simulink model "fft32kpt_ssr16_fixed"  (R2024b)
settings: Solver=VariableStepAuto  StartTime=0.0  StopTime=sample_period*N*5  RelTol=1e-3
PreLoadFcn:
  | clk_freq = 570e6; % PL clock frequency
  | sample_period = 1/(570e6*16); % 570Msps*16parallel paths
  | N=32768; % fft point size
  | binw=(1/sample_period) / 2*N; % bin width
  | 
  | bin_freq = 2*pi*11*binw+pi*binw; % sin, cos freq centering per channel
  | 
  | % for transpose block
  | DATA_WIDTH=16;
  | SSR=16;
  | M=16;
  | N1=N/M;
  | MEM_STYLE=4; % MEM OPTIONS: 4 - ULTRA, 0 - AUTO, 1 - BRAM, 5 - MIXED
InitFcn:
  | clk_freq = 570e6; % PL clock frequency
  | sample_period = 1/(570e6*16); % 570Msps*16parallel paths
  | N=32768; % fft point size
  | binw=(1/sample_period) / 2*N; % bin width
  | 
  | bin_freq = 2*pi*11*binw+pi*binw; % sin, cos freq centering per channel
  | 
  | % for transpose block
  | DATA_WIDTH=16;
  | SSR=16;
  | M=16;
  | N1=N/M;
  | MEM_STYLE=4; % MEM OPTIONS: 4 - ULTRA, 0 - AUTO, 1 - BRAM, 5 - MIXED
undefined symbols (not defined in the file or in its folder): None, S, vsva2197, xcvc1902
libraries: aieBasic x47, hdlBasic x39, aieUtilities x16, aieDSP x16, hdlUtilities x16, matrix_library x16, hdlSSR x13, simulink x1, dspxfrm3 x1, vmcUtilities x1
(part 1 of 3)
settings Model: Creator=mmi  LastModifiedBy=robg
settings DebuggingCC: UnconnectedInputMsg=warning  UnconnectedOutputMsg=warning  UnconnectedLineMsg=warning
settings HardwareCC: ProdBitPerPointer=32  ProdBitPerSizeT=32  ProdBitPerPtrDiffT=32  ProdLargestAtomicFloat=None  ProdIntDivRoundTo=Undefined  ProdEndianess=Unspecified  ProdWordSize=32  ProdHWDeviceType=ASIC/FPGA->ASIC/FPGA  TargetBitPerLong=64  TargetBitPerPointer=64  TargetBitPerSizeT=64  TargetBitPerPtrDiffT=64  TargetLongLongMode=on  TargetIntDivRoundTo=Zero  TargetEndianess=LittleEndian  TargetWordSize=64  TargetHWDeviceType=Custom Processor->MATLAB Host Computer  ProdEqTarget=off
settings ModelReferenceCC: EnableRefExpFcnMdlSchedulingChecks=on
settings RTWCC: GPUComputeCapability=3.5  DLArmComputeVersion=19.05
settings ConfigComp: CovBoundaryAbsTol=1.0e-5

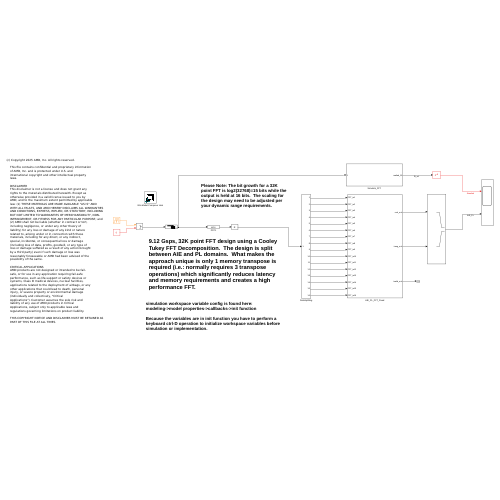
[thumbnail: Simulink's stored preview of the top-level diagram]
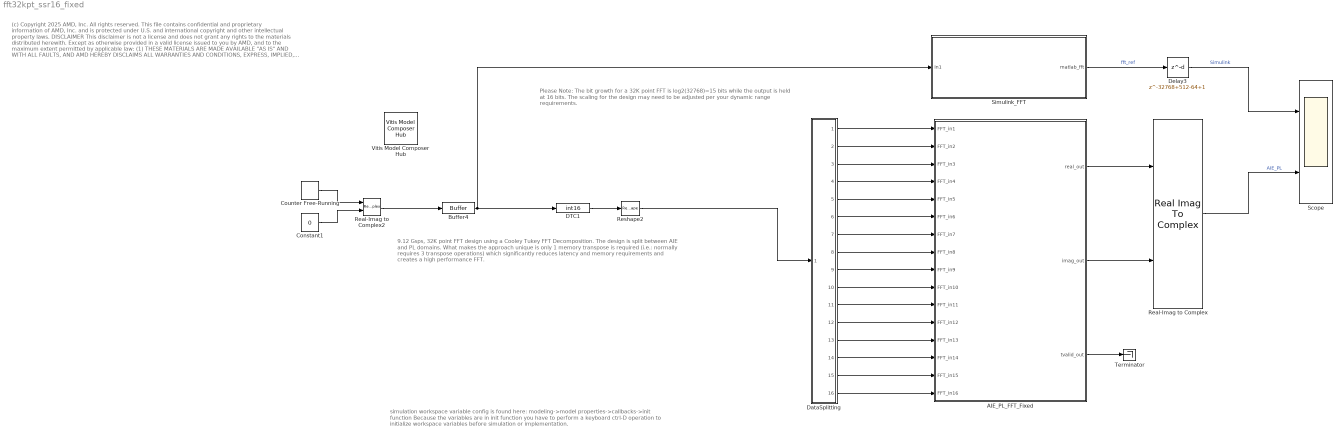
== system fft32kpt_ssr16_fixed ==
  note: simulation workspace variable config is found here:
      | modeling->model properties->callbacks->init function
      |
      | Because the variables are in init function you have to perform a keyboard ctrl-D operation to initialize workspace variables before simulation or implementation.
  note: 9.12 Gsps, 32K point FFT design using a Cooley Tukey FFT Decomposition. The design is split between AIE and PL domains. What makes the approach unique is only 1 memory transpose is required (i.e.: normally requires 3 transpose operations) which significantly reduces latency and memory requirements and creates a high performance FFT.
  note: Please Note: The bit growth for a 32K point FFT is log2(32768)=15 bits while the output is held at 16 bits. The scaling for the design may need to be adjusted per your dynamic range requirements.
  note: (c) Copyright 2025 AMD, Inc. All rights reserved.
      |
      | This file contains confidential and proprietary information
      | of AMD, Inc. and is protected under U.S. and
      | international copyright and other intellectual property
      | laws.
      |
      | DISCLAIMER
      | This disclaimer is not a license and does not grant any
      | rights to the materials distributed herewith. Except as
      | otherwise provided in a valid license issued to you by
      | AMD, and to the maximum extent permitted by applicable
      | law: (1) THESE MATERIALS ARE MADE AVAILABLE "AS IS" AND
      | WITH ALL FAULTS, AND AMD HEREBY DISCLAIMS ALL WARRANTIES
      | AND CONDITIONS, EXPRESS, IMPLIED, OR STATUTORY, INCLUDING
      | BUT NOT LIMITED TO WARRANTIES OF MERCHANTABILITY, NON-
      | INFRINGEMENT, OR FITNESS FOR ANY PARTICULAR PURPOSE; and
      | (2) AMD shall not be liable (whether in contract or tort,
      | including negligence, or under any other theory of
      | liability) for any loss or damage of any kind or nature
      | related to, arising under or in connection with these
      | materials, including for any direct, or any indirect,
      | special, incidental, or consequential loss or damage
      | (including loss of data, profits, goodwill, or any type of
      | loss or damage suffered as a result of any action brought
      | by a third party) even if such damage or loss was
      | reasonably foreseeable or AMD had been advised of the
      | possibility of the same.
      |
      | CRITICAL APPLICATIONS
      | AMD products are not designed or intended to be fail-
      | safe, or for use in any application requiring fail-safe
      | performance, such as life-support or safety devices or
      | systems, Class III medical devices, nuclear facilities,
      | applications related to the deployment of airbags, or any
      | other applications that could lead to death, personal
      | injury, or severe property or environmental damage
      | (individually and collectively, "Critical
      | Applications"). Customer assumes the sole risk and
      | liability of any use of AMD products in Critical
      | Applications, subject only to applicable laws and
      | regulations governing limitations on product liability.
      |
      | THIS COPYRIGHT NOTICE AND DISCLAIMER MUST BE RETAINED AS
      | PART OF THIS FILE AT ALL TIMES.
  AIE_PL_FFT_Fixed : Subsystem
  Buffer4 : Buffer  N=N  OutputFrames=off
  Constant1 : Constant  Value=0  OutDataTypeStr=Inherit: Inherit via back propagation  SampleTime=sample_period
  Counter Free-Running : simulink/Sources/Counter Free-Running  NumBits=log2(1024)  tsamp=sample_period
  DTC1 : DataTypeConversion  OutDataTypeStr=int16  SaturateOnIntegerOverflow=off  RndMeth=Floor
  DataSplitting : Subsystem
  Delay3 : Delay  DelayLength=32768+512-64+1
  Real-Imag to Complex : RealImagToComplex
  Real-Imag to Complex2 : RealImagToComplex
  Reshape2 : Reshape  OutputDimensionality=Customize  OutputDimensions=[16,N/16]
  Scope : Scope  NumInputPorts=2
  Simulink_FFT : Subsystem
  Terminator : Terminator
  Vitis Model Composer Hub : vmcUtilities/Vitis Model Composer Hub  Tag=genX  CodeGeneration=off  SubsystemName=AIE_2kFFT_cplxRot  BlockHierPath=fft32kpt_ssr16_fixed/AIE_PL_FFT_Fixed/AIE_2kFFT_cplxRot  CompilationType=VitisCompilation  SubsystemType=AIENode  ExportTypeV2=GenXO  StartColumn=1  NumberOfColumns=1  TargetDirectory=./code_FFT  exportDesign=off  analyzeDesign=on  validateDesignOnHw=off  ExportType=Vitis Subsystem  IpVendor=xilinx.com  IpLibrary=hls  IpVersion=1.0  IpHWLanguage=Verilog  AieCompilerOptions={}  AieSimulatorOptions={}  CreateTestbench=on  TestbenchStackSize=10  RunRtlSim=off  RunCSim=off  RunAieSim=on  AieSimTimeout=50000  RunAieSimProfiling=off  LaunchVitisAnalyzer=off  PlotOutput=off  RunX86Sim=off  X86SimTimeout=10  GenHwImage=off  GenLibadfXo=off  GenHwValidationCode=off  PlatformType=Specify Platform  Platform=/proj/xbuilds/SWIP/2024.2_1113_1001/installs/lin64/Vitis/2024.2/base_platforms/xilinx_vck190_base_202420_1/xilinx_vck190_base_202420_1.xpfm  HwSystemType=Baremetal  HwValidationTarget=hw  ProjDevice=Versal VCK190 Evaluation Platform (xcvc1902-vsva2197-2MP-e-S)  ProjDevicePart=xcvc1902-vsva2197-2MP-e-S  AIEType=AIE  SamplePeriod=-1  ClockFrequency=200  DataPathParallelism=1  xilinxfamily=versalaicore  part=xcvc1902  speed=-2MP-e-S  package=vsva2197  directory=./netlist_pl/ip/HDL_16ptFFT_tranpose/src  testbench=off  incr_netlist=off  synthesis_tool=Vivado  clock_wrapper=Clock Enables  dbl_ovrd=According to Block Masks  dcm_input_clock_period=10  sysclk_period=1e9/clk_freq  simulink_period=1/clk_freq  eval_field=0  IPInfoJsonString="{\"DUTSubsystemName\":\"AIE_2kFFT_cplxRot\",\"AIESubsystem\":{\"SubsystemName\":\"AIE_2kFFT_cplxRot\",\"TargetDirectory\":\"./code_FFT\",\"AIEArrayConfig\":\"Use entire AIE array\",\"StartColumn\":\"0\",\"NumberOfColumns\":\"1\"},\"SubsystemTag\":\"AIENode\"}"  LogFileName=/group/xcoswmktg2/robg/git/vmc_examples/github/Examples/AIENGINE_plus_PL/AIE_HDL/VersalFFT/code_FFT/model_composer.log  NThreads=4  IPConfigFile=/tmp/vmctmp-16428498816969006604/fft32kpt_ssr16_fixed_ipconfig.json
  wires:
  Buffer4/1 -> Simulink_FFT/1(In1), DTC1/1
  Constant1/1 -> Real-Imag to Complex2/2
  Counter Free-Running/1 -> Real-Imag to Complex2/1
  Real-Imag to Complex2/1 -> Buffer4/1
  DTC1/1 -> Reshape2/1
  Simulink_FFT/1(matlab_fft) -> Delay3/1  "fft_ref"
  Delay3/1 -> Scope/1  "Simulink"
  Reshape2/1 -> DataSplitting/1(In1)
  DataSplitting/1(Out1) -> AIE_PL_FFT_Fixed/1(FFT_in1)
  DataSplitting/2(Out2) -> AIE_PL_FFT_Fixed/2(FFT_in2)
  DataSplitting/3(Out3) -> AIE_PL_FFT_Fixed/3(FFT_in3)
  DataSplitting/4(Out4) -> AIE_PL_FFT_Fixed/4(FFT_in4)
  DataSplitting/5(Out5) -> AIE_PL_FFT_Fixed/5(FFT_in5)
  DataSplitting/6(Out6) -> AIE_PL_FFT_Fixed/6(FFT_in6)
  DataSplitting/7(Out7) -> AIE_PL_FFT_Fixed/7(FFT_in7)
  DataSplitting/8(Out8) -> AIE_PL_FFT_Fixed/8(FFT_in8)
  DataSplitting/9(Out9) -> AIE_PL_FFT_Fixed/9(FFT_in9)
  DataSplitting/10(Out10) -> AIE_PL_FFT_Fixed/10(FFT_in10)
  DataSplitting/11(Out11) -> AIE_PL_FFT_Fixed/11(FFT_in11)
  DataSplitting/12(Out12) -> AIE_PL_FFT_Fixed/12(FFT_in12)
  DataSplitting/13(Out13) -> AIE_PL_FFT_Fixed/13(FFT_in13)
  DataSplitting/14(Out14) -> AIE_PL_FFT_Fixed/14(FFT_in14)
  DataSplitting/15(Out15) -> AIE_PL_FFT_Fixed/15(FFT_in15)
  DataSplitting/16(Out16) -> AIE_PL_FFT_Fixed/16(FFT_in16)
  Real-Imag to Complex/1 -> Scope/2  "AIE_PL"
  AIE_PL_FFT_Fixed/2(imag_out) -> Real-Imag to Complex/2
  AIE_PL_FFT_Fixed/1(real_out) -> Real-Imag to Complex/1
  AIE_PL_FFT_Fixed/3(tvalid_out) -> Terminator/1

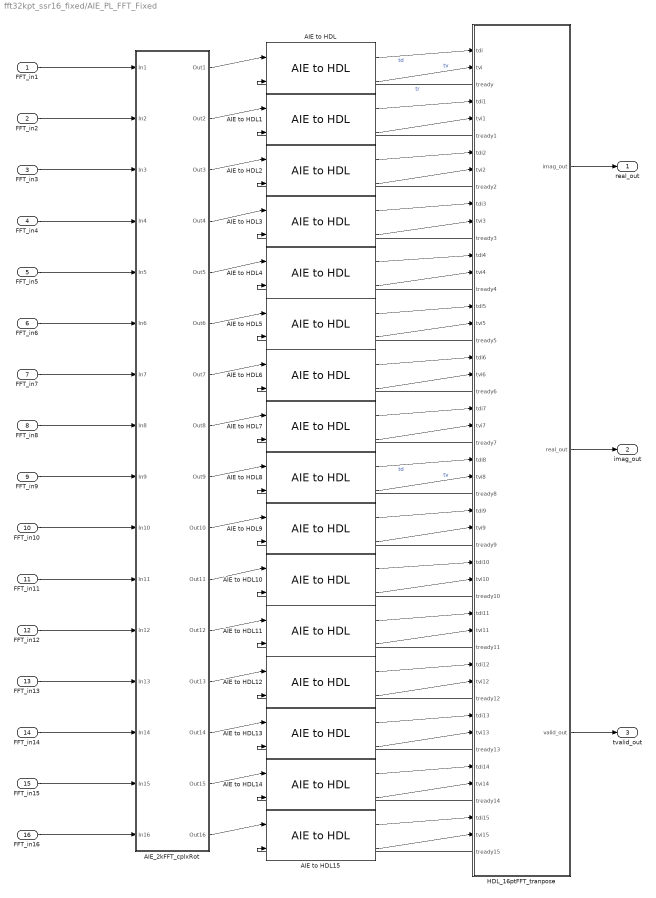
== system fft32kpt_ssr16_fixed/AIE_PL_FFT_Fixed ==
  FFT_in1 : Inport
  FFT_in2 : Inport  Port=2
  FFT_in3 : Inport  Port=3
  FFT_in4 : Inport  Port=4
  FFT_in5 : Inport  Port=5
  FFT_in6 : Inport  Port=6
  FFT_in7 : Inport  Port=7
  FFT_in8 : Inport  Port=8
  FFT_in9 : Inport  Port=9
  FFT_in10 : Inport  Port=10
  FFT_in11 : Inport  Port=11
  FFT_in12 : Inport  Port=12
  FFT_in13 : Inport  Port=13
  FFT_in14 : Inport  Port=14
  FFT_in15 : Inport  Port=15
  FFT_in16 : Inport  Port=16
  AIE to HDL{,1..15} (16 alike) : aieUtilities/AIE to HDL  OutDataType=uint32  OutSampleTime=Inherit: Same as tready
  AIE_2kFFT_cplxRot : Subsystem
  HDL_16ptFFT_tranpose : Subsystem
      settings: PortSchema="{\"entries\":[{\"content\":{\"sides\":[{\"content\":{\"connectorIds\":[\"In1\",\"In2\",\"Out4\",\"In3\",\"In4\",\"Out5\",\"In5\",\"In6\",\"Out6\",\"In7\",\"In8\",\"Out7\",\"In9\",\"In10\",\"Out8\",\"In11\",\"In12\",\"Out9\",\"In13\",\"In14\",\"Out10\",\"In15\",\"In16\",\"Out11\",\"In17\",\"In18\",\"Out12\",\"In19\",\"In20\",\"Out13\",\"In21\",\"In22\",\"Out14\",\"In23\",\"In24\",\"Out15\",\"In25\",\"In26\",\"Out16\",\"In27\",\"In28\",\"Out17\",\"In29\",\"In30\",\"Out18\",\"In31\",\"In32\",\"Out19\"]},\"type\":\"ConnectorPlacement.EquallySpacedRectSide\",\"uuid\":\"1fcf9dfd-1567-4542-995e-9e6658c7efa0\"},{\"content\":{\"connectorIds\":[\"Out1\",\"Out2\",\"Out3\"],\"side\":\"RIGHT\"},\"type\":\"ConnectorPlacement.EquallySpacedRectSide\",\"uuid\":\"6859206f-de88-49bd-8a59-387770ef842c\"},{\"content\":{\"side\":\"TOP\"},\"type\":\"ConnectorPlacement.EquallySpacedRectSide\",\"uuid\":\"208ed344-3d94-4bff-bef3-62ad006f8b17\"}]},\"type\":\"ConnectorPlacement.EquallySpacedConnector\",\"uuid\":\"de4bb24f-a4fa-4599-99f5-d3c88327bd77\"}],\"packageUris\":[\"http://schema.mathworks.com/mf0/Connector/R2020b\"],\"version\":\"1.0\"}"
  real_out : Outport
  imag_out : Outport  Port=2
  tvalid_out : Outport  Port=3
  wires:
  AIE_2kFFT_cplxRot/14(Out14) -> AIE to HDL13/1
  AIE_2kFFT_cplxRot/2(Out2) -> AIE to HDL1/1
  FFT_in3/1 -> AIE_2kFFT_cplxRot/3(In3)
  AIE_2kFFT_cplxRot/16(Out16) -> AIE to HDL15/1
  AIE_2kFFT_cplxRot/1(Out1) -> AIE to HDL/1
  AIE_2kFFT_cplxRot/3(Out3) -> AIE to HDL2/1
  AIE_2kFFT_cplxRot/15(Out15) -> AIE to HDL14/1
  AIE_2kFFT_cplxRot/5(Out5) -> AIE to HDL4/1
  AIE_2kFFT_cplxRot/7(Out7) -> AIE to HDL6/1
  FFT_in11/1 -> AIE_2kFFT_cplxRot/11(In11)
  AIE_2kFFT_cplxRot/13(Out13) -> AIE to HDL12/1
  FFT_in5/1 -> AIE_2kFFT_cplxRot/5(In5)
  FFT_in4/1 -> AIE_2kFFT_cplxRot/4(In4)
  AIE_2kFFT_cplxRot/12(Out12) -> AIE to HDL11/1
  AIE_2kFFT_cplxRot/8(Out8) -> AIE to HDL7/1
  FFT_in15/1 -> AIE_2kFFT_cplxRot/15(In15)
  FFT_in13/1 -> AIE_2kFFT_cplxRot/13(In13)
  FFT_in7/1 -> AIE_2kFFT_cplxRot/7(In7)
  AIE_2kFFT_cplxRot/10(Out10) -> AIE to HDL9/1
  FFT_in10/1 -> AIE_2kFFT_cplxRot/10(In10)
  FFT_in8/1 -> AIE_2kFFT_cplxRot/8(In8)
  FFT_in6/1 -> AIE_2kFFT_cplxRot/6(In6)
  FFT_in12/1 -> AIE_2kFFT_cplxRot/12(In12)
  FFT_in16/1 -> AIE_2kFFT_cplxRot/16(In16)
  FFT_in9/1 -> AIE_2kFFT_cplxRot/9(In9)
  FFT_in2/1 -> AIE_2kFFT_cplxRot/2(In2)
  FFT_in14/1 -> AIE_2kFFT_cplxRot/14(In14)
  AIE_2kFFT_cplxRot/9(Out9) -> AIE to HDL8/1
  AIE_2kFFT_cplxRot/11(Out11) -> AIE to HDL10/1
  AIE_2kFFT_cplxRot/4(Out4) -> AIE to HDL3/1
  AIE_2kFFT_cplxRot/6(Out6) -> AIE to HDL5/1
  FFT_in1/1 -> AIE_2kFFT_cplxRot/1(In1)
  AIE to HDL/2 -> HDL_16ptFFT_tranpose/2(tvi)  "tv"
  AIE to HDL/1 -> HDL_16ptFFT_tranpose/1(tdi)  "td"
  HDL_16ptFFT_tranpose/4(tready) -> AIE to HDL/2  "tr"
  AIE to HDL1/1 -> HDL_16ptFFT_tranpose/3(tdi1)
  AIE to HDL1/2 -> HDL_16ptFFT_tranpose/4(tvi1)
  HDL_16ptFFT_tranpose/5(tready1) -> AIE to HDL1/2
  HDL_16ptFFT_tranpose/6(tready2) -> AIE to HDL2/2
  AIE to HDL2/2 -> HDL_16ptFFT_tranpose/6(tvi2)
  AIE to HDL2/1 -> HDL_16ptFFT_tranpose/5(tdi2)
  AIE to HDL3/2 -> HDL_16ptFFT_tranpose/8(tvi3)
  HDL_16ptFFT_tranpose/7(tready3) -> AIE to HDL3/2
  AIE to HDL3/1 -> HDL_16ptFFT_tranpose/7(tdi3)
  HDL_16ptFFT_tranpose/8(tready4) -> AIE to HDL4/2
  AIE to HDL4/2 -> HDL_16ptFFT_tranpose/10(tvi4)
  AIE to HDL4/1 -> HDL_16ptFFT_tranpose/9(tdi4)
  AIE to HDL5/1 -> HDL_16ptFFT_tranpose/11(tdi5)
  AIE to HDL5/2 -> HDL_16ptFFT_tranpose/12(tvi5)
  HDL_16ptFFT_tranpose/9(tready5) -> AIE to HDL5/2
  AIE to HDL6/1 -> HDL_16ptFFT_tranpose/13(tdi6)
  AIE to HDL6/2 -> HDL_16ptFFT_tranpose/14(tvi6)
  HDL_16ptFFT_tranpose/10(tready6) -> AIE to HDL6/2
  HDL_16ptFFT_tranpose/11(tready7) -> AIE to HDL7/2
  AIE to HDL7/1 -> HDL_16ptFFT_tranpose/15(tdi7)
  AIE to HDL7/2 -> HDL_16ptFFT_tranpose/16(tvi7)
  AIE to HDL8/1 -> HDL_16ptFFT_tranpose/17(tdi8)  "td"
  AIE to HDL8/2 -> HDL_16ptFFT_tranpose/18(tvi8)  "tv"
  HDL_16ptFFT_tranpose/12(tready8) -> AIE to HDL8/2
  AIE to HDL9/1 -> HDL_16ptFFT_tranpose/19(tdi9)
  AIE to HDL9/2 -> HDL_16ptFFT_tranpose/20(tvi9)
  HDL_16ptFFT_tranpose/13(tready9) -> AIE to HDL9/2
  AIE to HDL10/1 -> HDL_16ptFFT_tranpose/21(tdi10)
  AIE to HDL10/2 -> HDL_16ptFFT_tranpose/22(tvi10)
  HDL_16ptFFT_tranpose/14(tready10) -> AIE to HDL10/2
  AIE to HDL11/1 -> HDL_16ptFFT_tranpose/23(tdi11)
  AIE to HDL11/2 -> HDL_16ptFFT_tranpose/24(tvi11)
  HDL_16ptFFT_tranpose/15(tready11) -> AIE to HDL11/2
  AIE to HDL12/1 -> HDL_16ptFFT_tranpose/25(tdi12)
  AIE to HDL12/2 -> HDL_16ptFFT_tranpose/26(tvi12)
  HDL_16ptFFT_tranpose/19(tready15) -> AIE to HDL15/2
  AIE to HDL15/2 -> HDL_16ptFFT_tranpose/32(tvi15)
  AIE to HDL15/1 -> HDL_16ptFFT_tranpose/31(tdi15)
  HDL_16ptFFT_tranpose/18(tready14) -> AIE to HDL14/2
  AIE to HDL14/2 -> HDL_16ptFFT_tranpose/30(tvi14)
  AIE to HDL14/1 -> HDL_16ptFFT_tranpose/29(tdi14)
  HDL_16ptFFT_tranpose/17(tready13) -> AIE to HDL13/2
  AIE to HDL13/1 -> HDL_16ptFFT_tranpose/27(tdi13)
  AIE to HDL13/2 -> HDL_16ptFFT_tranpose/28(tvi13)
  HDL_16ptFFT_tranpose/16(tready12) -> AIE to HDL12/2
  HDL_16ptFFT_tranpose/1(imag_out) -> real_out/1
  HDL_16ptFFT_tranpose/2(real_out) -> imag_out/1
  HDL_16ptFFT_tranpose/3(valid_out) -> tvalid_out/1

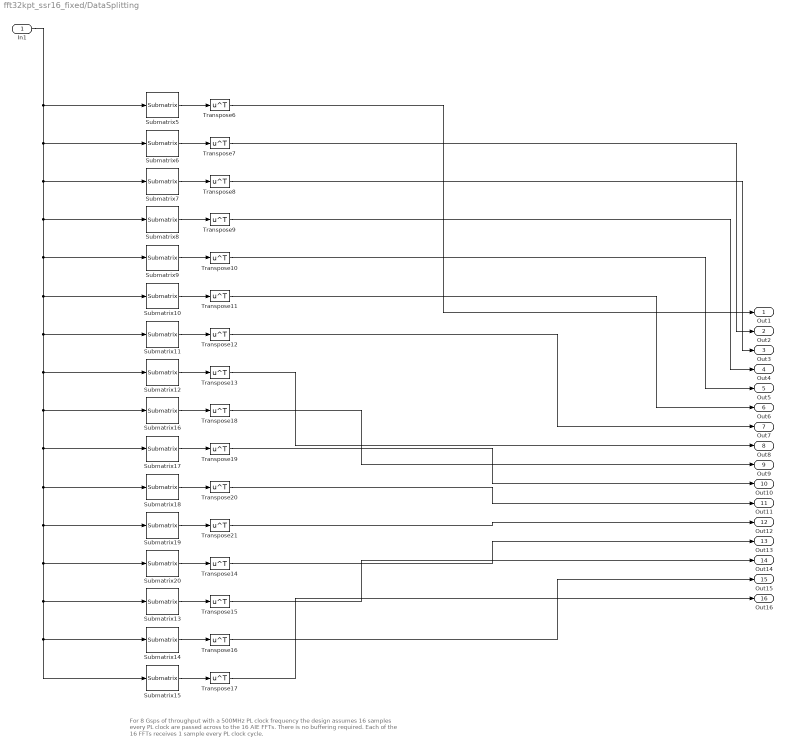
== system fft32kpt_ssr16_fixed/DataSplitting ==
  note: For 8 Gsps of throughput with a 500MHz PL clock frequency the design assumes 16 samples every PL clock are passed across to the 16 AIE FFTs.
      |
      | There is no buffering required. Each of the 16 FFTs receives 1 sample every PL clock cycle.
  In1 : Inport
  Submatrix10 : matrix_library/Submatrix  RowSpan=One row  RowStartMode=Index  RowStartIndex=6  RowEndMode=Last  RowEndIndex=1  ColSpan=Range of columns  ColStartMode=First  ColStartIndex=1  ColEndMode=Last  ColEndIndex=1
  Submatrix11 : matrix_library/Submatrix  RowSpan=One row  RowStartMode=Index  RowStartIndex=7  RowEndMode=Last  RowEndIndex=1  ColSpan=Range of columns  ColStartMode=First  ColStartIndex=1  ColEndMode=Last  ColEndIndex=1
  Submatrix12 : matrix_library/Submatrix  RowSpan=One row  RowStartMode=Index  RowStartIndex=8  RowEndMode=Last  RowEndIndex=1  ColSpan=Range of columns  ColStartMode=First  ColStartIndex=1  ColEndMode=Last  ColEndIndex=1
  Submatrix13 : matrix_library/Submatrix  RowSpan=One row  RowStartMode=Index  RowStartIndex=14  RowEndMode=Last  RowEndIndex=1  ColSpan=Range of columns  ColStartMode=First  ColStartIndex=1  ColEndMode=Last  ColEndIndex=1
  Submatrix14 : matrix_library/Submatrix  RowSpan=One row  RowStartMode=Index  RowStartIndex=15  RowEndMode=Last  RowEndIndex=1  ColSpan=Range of columns  ColStartMode=First  ColStartIndex=1  ColEndMode=Last  ColEndIndex=1
  Submatrix15 : matrix_library/Submatrix  RowSpan=One row  RowStartMode=Index  RowStartIndex=16  RowEndMode=Last  RowEndIndex=1  ColSpan=Range of columns  ColStartMode=First  ColStartIndex=1  ColEndMode=Last  ColEndIndex=1
  Submatrix16 : matrix_library/Submatrix  RowSpan=One row  RowStartMode=Index  RowStartIndex=9  RowEndMode=Last  RowEndIndex=1  ColSpan=Range of columns  ColStartMode=First  ColStartIndex=1  ColEndMode=Last  ColEndIndex=1
  Submatrix17 : matrix_library/Submatrix  RowSpan=One row  RowStartMode=Index  RowStartIndex=10  RowEndMode=Last  RowEndIndex=1  ColSpan=Range of columns  ColStartMode=First  ColStartIndex=1  ColEndMode=Last  ColEndIndex=1
  Submatrix18 : matrix_library/Submatrix  RowSpan=One row  RowStartMode=Index  RowStartIndex=11  RowEndMode=Last  RowEndIndex=1  ColSpan=Range of columns  ColStartMode=First  ColStartIndex=1  ColEndMode=Last  ColEndIndex=1
  Submatrix19 : matrix_library/Submatrix  RowSpan=One row  RowStartMode=Index  RowStartIndex=12  RowEndMode=Last  RowEndIndex=1  ColSpan=Range of columns  ColStartMode=First  ColStartIndex=1  ColEndMode=Last  ColEndIndex=1
  Submatrix20 : matrix_library/Submatrix  RowSpan=One row  RowStartMode=Index  RowStartIndex=13  RowEndMode=Last  RowEndIndex=1  ColSpan=Range of columns  ColStartMode=First  ColStartIndex=1  ColEndMode=Last  ColEndIndex=1
  Submatrix5 : matrix_library/Submatrix  RowSpan=One row  RowStartMode=First  RowStartIndex=1  RowEndMode=Last  RowEndIndex=1  ColSpan=Range of columns  ColStartMode=First  ColStartIndex=1  ColEndMode=Last  ColEndIndex=1
  Submatrix6 : matrix_library/Submatrix  RowSpan=One row  RowStartMode=Index  RowStartIndex=2  RowEndMode=Last  RowEndIndex=1  ColSpan=Range of columns  ColStartMode=First  ColStartIndex=1  ColEndMode=Last  ColEndIndex=1
  Submatrix7 : matrix_library/Submatrix  RowSpan=One row  RowStartMode=Index  RowStartIndex=3  RowEndMode=Last  RowEndIndex=1  ColSpan=Range of columns  ColStartMode=First  ColStartIndex=1  ColEndMode=Last  ColEndIndex=1
  Submatrix8 : matrix_library/Submatrix  RowSpan=One row  RowStartMode=Index  RowStartIndex=4  RowEndMode=Last  RowEndIndex=1  ColSpan=Range of columns  ColStartMode=First  ColStartIndex=1  ColEndMode=Last  ColEndIndex=1
  Submatrix9 : matrix_library/Submatrix  RowSpan=One row  RowStartMode=Index  RowStartIndex=5  RowEndMode=Last  RowEndIndex=1  ColSpan=Range of columns  ColStartMode=First  ColStartIndex=1  ColEndMode=Last  ColEndIndex=1
  Transpose{6..21} (16 alike) : Math  Operator=transpose
  Out1 : Outport
  Out2 : Outport  Port=2
  Out3 : Outport  Port=3
  Out4 : Outport  Port=4
  Out5 : Outport  Port=5
  Out6 : Outport  Port=6
  Out7 : Outport  Port=7
  Out8 : Outport  Port=8
  Out9 : Outport  Port=9
  Out10 : Outport  Port=10
  Out11 : Outport  Port=11
  Out12 : Outport  Port=12
  Out13 : Outport  Port=13
  Out14 : Outport  Port=14
  Out15 : Outport  Port=15
  Out16 : Outport  Port=16
  wires:
  Transpose10/1 -> Out5/1
  Transpose7/1 -> Out2/1
  Transpose6/1 -> Out1/1
  Submatrix12/1 -> Transpose13/1
  Submatrix20/1 -> Transpose14/1
  Transpose11/1 -> Out6/1
  Transpose14/1 -> Out13/1
  Submatrix18/1 -> Transpose20/1
  Submatrix17/1 -> Transpose19/1
  Submatrix7/1 -> Transpose8/1
  Transpose9/1 -> Out4/1
  Submatrix6/1 -> Transpose7/1
  Submatrix5/1 -> Transpose6/1
  Transpose20/1 -> Out11/1
  Submatrix9/1 -> Transpose10/1
  Submatrix16/1 -> Transpose18/1
  Submatrix8/1 -> Transpose9/1
  Submatrix14/1 -> Transpose16/1
  Submatrix11/1 -> Transpose12/1
  Submatrix10/1 -> Transpose11/1
  Transpose12/1 -> Out7/1
  Transpose13/1 -> Out8/1
  Transpose18/1 -> Out9/1
  In1/1 -> Submatrix14/1, Submatrix15/1, Submatrix13/1, Submatrix20/1, Submatrix19/1, Submatrix18/1, Submatrix17/1, Submatrix16/1, Submatrix12/1, Submatrix11/1, Submatrix10/1, Submatrix9/1, Submatrix8/1, Submatrix7/1, Submatrix6/1, Submatrix5/1
  Submatrix19/1 -> Transpose21/1
  Transpose16/1 -> Out15/1
  Transpose8/1 -> Out3/1
  Transpose17/1 -> Out16/1
  Transpose21/1 -> Out12/1
  Submatrix15/1 -> Transpose17/1
  Submatrix13/1 -> Transpose15/1
  Transpose19/1 -> Out10/1
  Transpose15/1 -> Out14/1

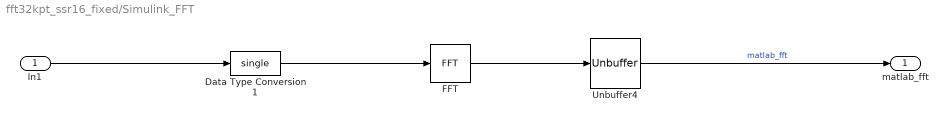
== system fft32kpt_ssr16_fixed/Simulink_FFT ==
  In1 : Inport
  Data Type Conversion1 : DataTypeConversion  OutDataTypeStr=single  SaturateOnIntegerOverflow=off  RndMeth=Floor
  FFT : dspxfrm3/FFT  FFTImplementation=Auto  CompMethod=Table lookup  TableOpt=NEW  TableOptActive=Speed  BitRevOrder=off  Normalize=on  InheritFFTLength=on  FFTLength=64  WrapInput=on  roundingMode=Floor  overflowMode=off  firstCoeffDataTypeStr=Inherit: Same word length as input  firstCoeffLastDataTypeStr=Inherit: Same word length as input  outputMin=[]  outputMax=[]
  Unbuffer4 : Unbuffer
  matlab_fft : Outport
  wires:
  Data Type Conversion1/1 -> FFT/1
  FFT/1 -> Unbuffer4/1
  In1/1 -> Data Type Conversion1/1
  Unbuffer4/1 -> matlab_fft/1  "matlab_fft"
